simulink model "w2problem1"  (R2020b)
settings: Solver=VariableStepAuto  StartTime=0.0  StopTime=300  RelTol=1e-3
settings Model: Creator=k.Raviteja  LastModifiedBy=k.Raviteja

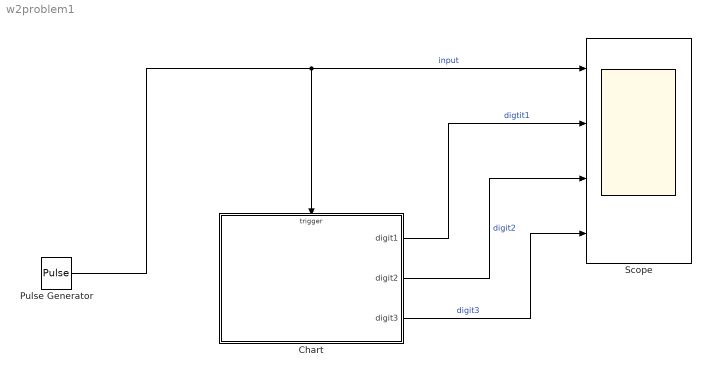
== system w2problem1 ==
  Chart : Stateflow chart  TreatAsAtomicUnit=on
  Pulse Generator : DiscretePulseGenerator  PulseType=Time based  Amplitude=2  Period=1  PulseWidth=50
  Scope : Scope  NumInputPorts=4
  wires:
  Chart/3(digit3) -> Scope/4  "digit3"
  Chart/2(digit2) -> Scope/3  "digit2"
  Chart/1(digit1) -> Scope/2  "digtit1"
  Pulse Generator/1 -> Chart/Trigger, Scope/1  "input"

== stateflow chart w2problem1/Chart ==
  settings: executeAtInitialization=1
  state Firstdigit [parallel]
    settings: executionOrder=1
    state a
      entry:
      digit1=0;
    state b
      entry:
      digit1=1;
    state c
      entry:
      digit1=2;
    state d
      entry:
      digit1=3;
    state e
      entry:
      digit1=4;
    state f
      entry:
      digit1=5;
    (default) -> Firstdigit.a
    Firstdigit.f -> Firstdigit.a : x/{Seconddigit.y}
    Firstdigit.a -> Firstdigit.b : x
    Firstdigit.b -> Firstdigit.c : x
    Firstdigit.c -> Firstdigit.d : x
    Firstdigit.d -> Firstdigit.e : x
    Firstdigit.e -> Firstdigit.f : x
  state Seconddigit [parallel]
    settings: executionOrder=2
    state a
      entry:
      digit2=0;
    state b
      entry:
      digit2=1;
    state c
      entry:
      digit2=2;
    state d
      entry:
      digit2=3;
    state e
      entry:
      digit2=4;
    state f
      entry:
      digit2=5;
    (default) -> Seconddigit.a
    Seconddigit.f -> Seconddigit.a : y/{Thirddigt.z}
    Seconddigit.a -> Seconddigit.b : y
    Seconddigit.b -> Seconddigit.c : y
    Seconddigit.c -> Seconddigit.d : y
    Seconddigit.d -> Seconddigit.e : y
    Seconddigit.e -> Seconddigit.f : y
  state Thirddigt [parallel]
    settings: executionOrder=3
    state a
      entry:
      digit3=0;
    state b
      entry:
      digit3=1;
    state c
      entry:
      digit3=2;
    state d
      entry:
      digit3=3;
    state e1
      entry:
      digit3=4;
    state f
      entry:
      digit3=5;
    (default) -> Thirddigt.a
    Thirddigt.f -> Thirddigt.a : z
    Thirddigt.a -> Thirddigt.b : z
    Thirddigt.b -> Thirddigt.c : z
    Thirddigt.c -> Thirddigt.d : z
    Thirddigt.d -> e1 : z
    e1 -> Thirddigt.f : z
  data: digit1 output; digit2 output; digit3 output
  events: y local RISING_EDGE_EVENT; z local RISING_EDGE_EVENT; x input RISING_EDGE_EVENT
